simulink model "Taylor_Servo"  (R2021a)
settings: Solver=ode45  StartTime=0.0  StopTime=20  MaxStep=params.maxStepSize  RelTol=1e-3
undefined symbols (not defined in the file): C, F1, F2, maxW, params, y_d, z_d
settings Model: Creator=Sopagna  LastModifiedBy=sarmiento
settings SolverCC: AlgebraicLoopSolver=LineSearch
settings DebuggingCC: SFMachineParentedDataDiag=warning

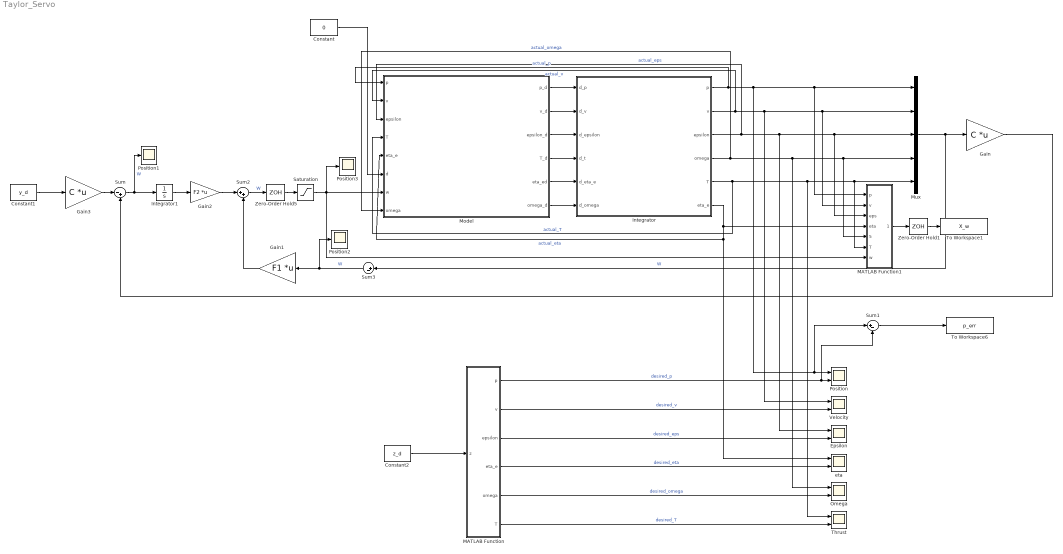
== system Taylor_Servo ==
  Constant : Constant  Value=0
  Constant1 : Constant  Value=y_d
  Constant2 : Constant  Value=z_d
  Epsilon : Scope  NumInputPorts=2
  Gain : Gain  Gain=C  Multiplication=Matrix(K*u) (u vector)
  Gain1 : Gain  Gain=F1  Multiplication=Matrix(K*u) (u vector)
  Gain2 : Gain  Gain=F2  Multiplication=Matrix(K*u) (u vector)
  Gain3 : Gain  Gain=C  Multiplication=Matrix(K*u) (u vector)
  Integrator : Subsystem
  Integrator1 : Integrator
  MATLAB Function : MATLAB Function  TreatAsAtomicUnit=on
  MATLAB Function1 : MATLAB Function  TreatAsAtomicUnit=on
  Model : MATLAB Function  TreatAsAtomicUnit=on
  Mux : Mux  Inputs=5
  Omega : Scope  NumInputPorts=2
  Position : Scope  NumInputPorts=2
  Position1 : Scope
  Position2 : Scope
  Position3 : Scope
  Saturation : Saturate  UpperLimit=maxW  LowerLimit=-maxW
  Sum : Sum  Inputs=|-+
  Sum1 : Sum  Inputs=|+-
  Sum2 : Sum  Inputs=|++
  Sum3 : Sum  Inputs=|+-
  Thrust : Scope  NumInputPorts=2
  To Workspace1 : ToWorkspace  VariableName=X_w  SampleTime=-1
      settings: Save2DSignal=2-D array (concatenate along first dimension)
  To Workspace6 : ToWorkspace  VariableName=p_err  SampleTime=-1
      settings: Save2DSignal=2-D array (concatenate along first dimension)
  Velocity : Scope  NumInputPorts=2
  Zero-Order Hold1 : ZeroOrderHold  SampleTime=params.ST_id
  Zero-Order Hold5 : ZeroOrderHold  SampleTime=params.ST_id
  eta : Scope  NumInputPorts=2
  wires:
  Model/5(eta_ed) -> Integrator/5(d_eta_e)
  Constant/1 -> Model/6(d)
  Model/1(p_d) -> Integrator/1(d_p)
  Model/2(v_d) -> Integrator/2(d_v)
  Model/3(epsilon_d) -> Integrator/3(d_epsilon)
  Model/4(T_d) -> Integrator/4(d_t)
  Model/6(omega_d) -> Integrator/6(d_omega)
  MATLAB Function/1(p) -> Sum1/2, Position/2  "desired_p"
  MATLAB Function/2(v) -> Velocity/2  "desired_v"
  MATLAB Function/3(epsilon) -> Epsilon/2  "desired_eps"
  MATLAB Function/4(eta_e) -> eta/2  "desired_eta"
  Sum1/1 -> To Workspace6/1
  MATLAB Function/5(omega) -> Omega/2  "desired_omega"
  MATLAB Function/6(T) -> Thrust/2  "desired_T"
  Sum/1 -> Position1/1, Integrator1/1  "W"
  Gain1/1 -> Sum2/2
  Integrator1/1 -> Gain2/1
  Constant2/1 -> MATLAB Function/1(z)
  Mux/1 -> Sum3/1, Gain/1  "W"
  Sum3/1 -> Position2/1, Gain1/1  "W"
  Gain2/1 -> Sum2/1
  Saturation/1 -> MATLAB Function1/7(w), Model/7(w), Position3/1
  Zero-Order Hold5/1 -> Saturation/1
  Sum2/1 -> Zero-Order Hold5/1  "W"
  Gain3/1 -> Sum/1
  Constant1/1 -> Gain3/1
  Integrator/1(p) -> Model/1(p), Sum1/1, Position/1, MATLAB Function1/1(p), Mux/1  "actual_p"
  Integrator/2(v) -> Model/2(v), Velocity/1, MATLAB Function1/2(v), Mux/2  "actual_v"
  Integrator/3(epsilon) -> Model/3(epsilon), Epsilon/1, MATLAB Function1/3(eps), Mux/3  "actual_eps"
  Integrator/4(omega) -> Model/8(omega), Omega/1, MATLAB Function1/5(omega), Mux/4  "actual_omega"
  Integrator/5(T) -> Model/4(T), Thrust/1, MATLAB Function1/6(T), Mux/5  "actual_T"
  Integrator/6(eta_e) -> MATLAB Function1/4(eta), eta/1, Model/5(eta_e)  "actual_eta"
  Gain/1 -> Sum/2
  MATLAB Function1/1(X_w) -> Zero-Order Hold1/1
  Zero-Order Hold1/1 -> To Workspace1/1

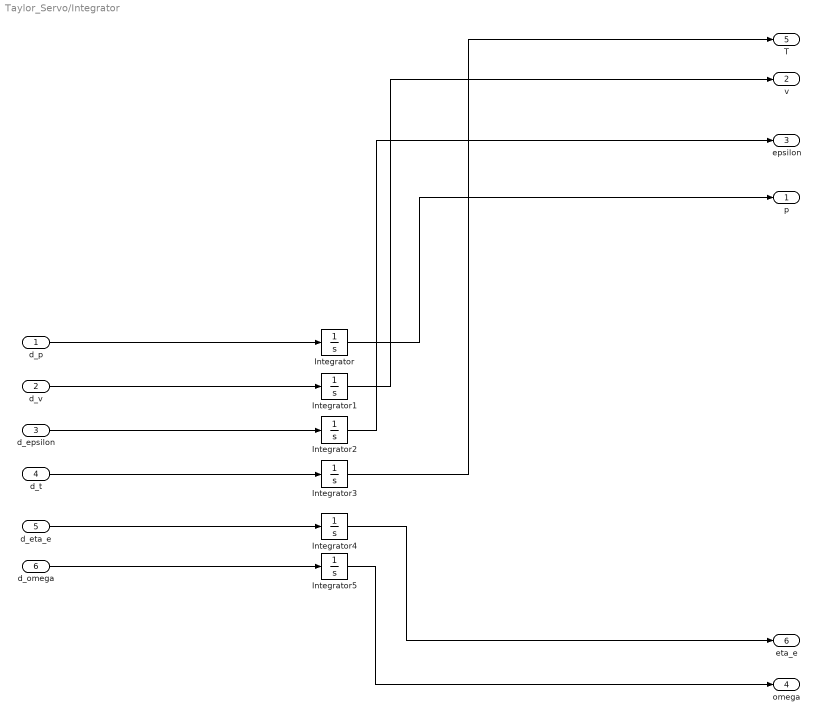
== system Taylor_Servo/Integrator ==
  d_p : Inport
  d_v : Inport  Port=2
  d_epsilon : Inport  Port=3
  d_t : Inport  Port=4
  d_eta_e : Inport  Port=5
  d_omega : Inport  Port=6
  Integrator : Integrator  InitialCondition=params.p_0
  Integrator1 : Integrator  InitialCondition=params.v_0
  Integrator2 : Integrator  InitialCondition=params.epsilon_0
  Integrator3 : Integrator  InitialCondition=params.T_0
  Integrator4 : Integrator  InitialCondition=params.eta_e0
  Integrator5 : Integrator  InitialCondition=params.omega_0
  p : Outport
  v : Outport  Port=2
  epsilon : Outport  Port=3
  omega : Outport  Port=4
  T : Outport  Port=5
  eta_e : Outport  Port=6
  wires:
  d_eta_e/1 -> Integrator4/1
  d_epsilon/1 -> Integrator2/1
  d_p/1 -> Integrator/1
  Integrator2/1 -> epsilon/1
  Integrator/1 -> p/1
  Integrator1/1 -> v/1
  d_t/1 -> Integrator3/1
  Integrator3/1 -> T/1
  d_v/1 -> Integrator1/1
  Integrator4/1 -> eta_e/1
  d_omega/1 -> Integrator5/1
  Integrator5/1 -> omega/1

== matlab function Taylor_Servo/MATLAB Function1 ==
  data: p input; X_w output; v input; eps input; eta input; omega input; T input; w input
function X_w = fcn(p, v, eps, eta, omega, T, w)

X_w = [p; v; eps; eta; omega; T; w];

== matlab function Taylor_Servo/Model ==
  data: p input size=[3 1]; v input size=[3 1]; epsilon input size=[3 1]; T input size=1; eta_e input size=1; d input size=1; w input size=[4 1]; p_d output size=[3 1]; v_d output size=[3 1]; epsilon_d output size=[3 1]; T_d output size=1; eta_ed output size=1; omega_d output; omega input
function [p_d,v_d,epsilon_d,T_d,eta_ed, omega_d] = fnc_training(p,v,epsilon,T,eta_e,d,w, omega)
% function [p_d,v_d,epsilon_d,T_d,eta_ed, omega_d] = fnc_training(p,v,epsilon,T,eta_e,d,w)
%==========================Input Variable================================
w1 = w(1:3); 
w2 = w(4); % Total Thrust
g = 9.81; % Gravity

%==========================Equation of Motion============================
p_d = v;    %Velocity

%Aerodynamic Damping Coefficient
% K1 = 1;K2 = 1;K3 = 1; %Ns/m
% F_aero = [K1*v(1);K2*v(2);K3*v(3)];
F_dis = [2.50;1.25;2];
v_d = r_z(epsilon,eta_e,d)*T+[0;0;-g] + 1 * F_dis; %Acceleration

%==========================First Way to get euler para derivative========
% epsilon_d = w1; %1st time derivative of euler parameters
% eta_e = sqrt(1-epsilon'*epsilon); % Angle of rotation

%==========================Second Way to get euler para derivative========
K =0.5;
euler = [epsilon;
        eta_e];
C = euler.'*euler-1;
J_E = J(euler);
% omega = 2*inv(J_E(1:3,:))*w1;
e_d = 0.5 *J_E* omega -K*C*euler;
epsilon_d = e_d(1:3);
eta_ed = e_d(4);
omega_d = w1;

T_d = w2; %Time derivative of total thrust

== matlab function Taylor_Servo/MATLAB Function ==
  data: z input; p output; v output; epsilon output; eta_e output; omega output; T output
function [p, v, epsilon, eta_e, omega, T] = fcn(z)
p = z(1:3);
v = z(4:6);
epsilon = z(7:9);
eta_e = z(10);
omega = z(11:13);
T = z(14);
